simulink model "sm_ik_trajectory_model_horst"  (R2022b)
settings: Solver=FixedStepAuto  StartTime=0.0  StopTime=simtime  FixedStep=simtime/1000  RelTol=1e-3
values from neighbouring files (symbols this model uses):
  simtime = 1    [InverseKinematik_Horst.m]
undefined symbols (not defined in the file or in its folder): Angle, Axis, Levenberg, Marquardt
libraries: simulink x3, robotcorelib x1, robotmaniplib x1
settings Model: Creator=The MathWorks, Inc.  LastModifiedBy=ivo
settings SolverCC: AlgebraicLoopSolver=TrustRegion
settings DataIOCC: ReturnWorkspaceOutputs=off
settings DebuggingCC: UnconnectedInputMsg=warning  UnconnectedOutputMsg=warning  UnconnectedLineMsg=warning  SFMachineParentedDataDiag=warning  ArithmeticOperatorsInVariantConditions=warning
settings ModelReferenceCC: EnableRefExpFcnMdlSchedulingChecks=on
settings SFSimCC: SimUseLocalCustomCode=off  CustomCodeUndefinedFunction=UseInterfaceOnly
settings RTWCC: RTWUseLocalCustomCode=off

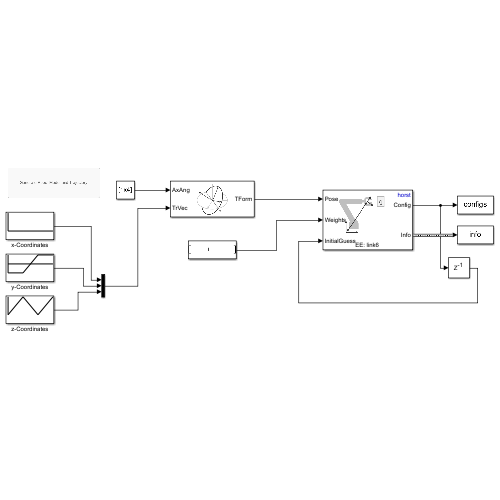
[thumbnail: Simulink's stored preview of the top-level diagram]
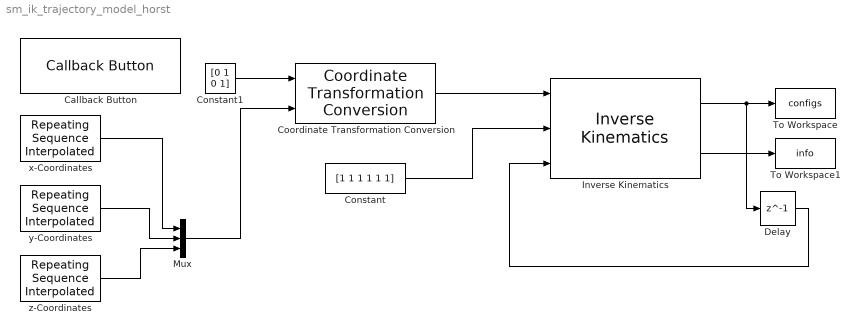
== system sm_ik_trajectory_model_horst ==
  Callback Button : CallbackButton  ButtonText=Generate Robot Model and Trajectory
      settings: ClickFcn=|
      | robot = importrobot('iiwa14.urdf');
      | robot.DataFormat = 'column';
      | x = 0.5*zeros(1,4)+0.25;
      | y = 0.25*[-1 -1 1 1];
      | z = 0.25*[-1 1 -1 1] + 0.75;
  Constant : Constant  Value=[1 1 1 1 1 1]
  Constant1 : Constant  Value=[0 1 0 1]  SampleTime=simtime/1000
  Coordinate Transformation Conversion : robotcorelib/Coordinate Transformation Conversion  InputRepresentation=Axis-Angle  InputEulerSequence=ZYX  ShowTrVecInputPort=on  OutputRepresentation=Homogeneous Transformation  OutputEulerSequence=ZYX  ShowTrVecOutputPort=on  SimulateUsing=Interpreted execution
  Delay : Delay  DelayLength=1  InitialCondition=ones(6,1)*10^-5
  Inverse Kinematics : robotmaniplib/Inverse Kinematics  RigidBodyTree=horst  EndEffector=link6  ShowInfo=on  SolverName=Levenberg-Marquardt  EnforceJointLimits=on  MaxIterations=1500  MaxTime=10  GradientTolerance=1e-7  SolutionTolerance=1e-6  StepTolerance=1e-14  ErrorChangeTolerance=1e-12  UseErrorDamping=on  DampingBias=0.0025  SimulateUsing=Interpreted execution
  Mux : Mux  Inputs=3
  To Workspace : ToWorkspace  VariableName=configs  SaveFormat=Timeseries  SampleTime=-1
  To Workspace1 : ToWorkspace  VariableName=info  SaveFormat=Timeseries  SampleTime=-1
  "x-Coordinates " : simulink/Sources/Repeating Sequence Interpolated  OutValues=x  TimeValues=timevector  LookUpMeth=Interpolation-Use End Values  tsamp=simtime/1000  OutMin=[]  OutMax=[]  OutDataTypeStr=double  OutputDataTypeScalingMode=double  OutDataType=fixdt(0,8)  OutScaling=2^-10
  y-Coordinates : simulink/Sources/Repeating Sequence Interpolated  OutValues=y  TimeValues=timevector  LookUpMeth=Interpolation-Use End Values  tsamp=simtime/1000  OutMin=[]  OutMax=[]  OutDataTypeStr=double  OutputDataTypeScalingMode=double  OutDataType=fixdt(0,8)  OutScaling=2^-10
  z-Coordinates : simulink/Sources/Repeating Sequence Interpolated  OutValues=z  TimeValues=timevector  LookUpMeth=Interpolation-Use End Values  tsamp=simtime/1000  OutMin=[]  OutMax=[]  OutDataTypeStr=double  OutputDataTypeScalingMode=double  OutDataType=fixdt(0,8)  OutScaling=2^-10
  wires:
  "x-Coordinates "/1 -> Mux/1
  Coordinate Transformation Conversion/1 -> Inverse Kinematics/1
  Mux/1 -> Coordinate Transformation Conversion/2
  y-Coordinates/1 -> Mux/2
  z-Coordinates/1 -> Mux/3
  Constant/1 -> Inverse Kinematics/2
  Inverse Kinematics/1 -> Delay/1, To Workspace/1
  Inverse Kinematics/2 -> To Workspace1/1
  Delay/1 -> Inverse Kinematics/3
  Constant1/1 -> Coordinate Transformation Conversion/1
